simulink model "Nyquist"  (R2016b)
settings: Solver=VariableStepAuto  StartTime=0.0  StopTime=30/1000  RelTol=1e-3
libraries: dsparch4 x1, commrandsrc3 x1, commsink2 x1, commsrccod2 x1
settings Model: Creator=white  LastModifiedBy=white

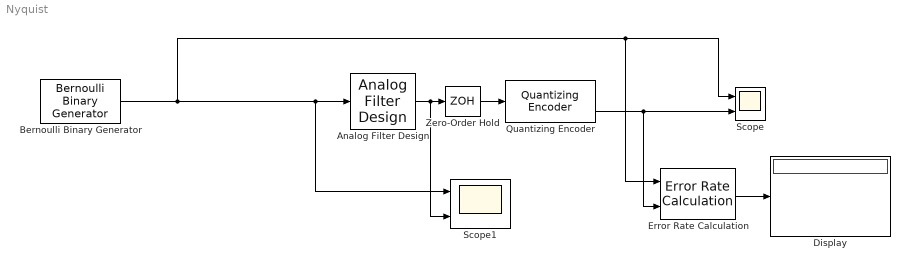
== system Nyquist ==
  Analog Filter Design : dsparch4/Analog Filter Design  method=Butterworth  filttype=Lowpass  N=6  Wlo=2*pi*1500  Whi=80  Rp=2  Rs=40
  Bernoulli Binary Generator : commrandsrc3/Bernoulli Binary Generator  ProbabilityOfZero=0.5  SeedSource=Auto  Seed=0  SampleTime=1/1000  SamplesPerFrame=1  OutputDataType=double  SimulateUsing=Interpreted execution
  Display : Display
  Error Rate Calculation : commsink2/Error Rate Calculation  N=1  st_delay=0  cp_mode=Entire frame  subframe=[]  PMode=Port  WsName=ErrorVec  RsMode2=off  stop=off  numErr=100  maxBits=1e6
  Quantizing Encoder : commsrccod2/Quantizing Encoder  partition=[0.5]  codebook=[0,1]  idxDType=double
  Scope : Scope  NumInputPorts=2
  Scope1 : Scope  NumInputPorts=2
  Zero-Order Hold : ZeroOrderHold  SampleTime=1/1000
  wires:
  Analog Filter Design/1 -> Scope1/2, Zero-Order Hold/1
  Zero-Order Hold/1 -> Quantizing Encoder/1
  Quantizing Encoder/2 -> Error Rate Calculation/2, Scope/2
  Error Rate Calculation/1 -> Display/1
  Bernoulli Binary Generator/1 -> Scope1/1, Analog Filter Design/1, Error Rate Calculation/1, Scope/1
